simulink model "quad_copter_ct_dt"  (R2016a)
settings: Solver=VariableStepAuto  StartTime=0.0  StopTime=10.0  RelTol=1e-3
undefined symbols (not defined in the file): DiscIntNeverNeededParam, Mixer, PitchRateModel_dt, PitchRateModel_tf, Ri_dt, Ri_tf, Ro_dt, Ro_tf, Ts
settings Model: Creator=tibo  LastModifiedBy=tibo

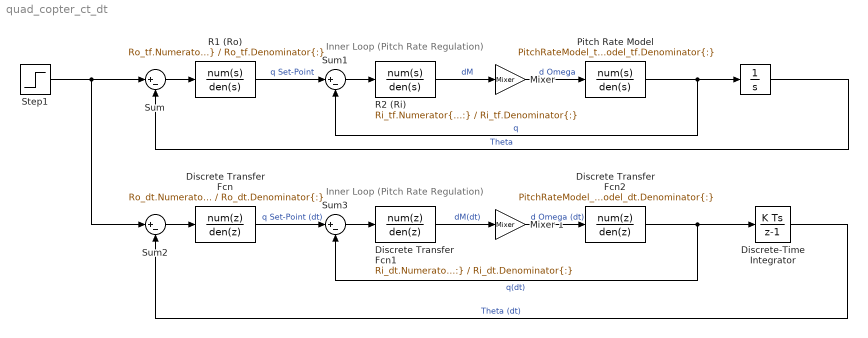
== system quad_copter_ct_dt ==
  note: Inner Loop (Pitch Rate Regulation)
  note: Inner Loop (Pitch Rate Regulation)
  " " : Integrator  ContinuousStateAttributes='PitchAngle'
  Discrete Transfer Fcn : DiscreteTransferFcn  Numerator=Ro_dt.Numerator{:}  Denominator=Ro_dt.Denominator{:}  SampleTime=Ts
  Discrete Transfer Fcn1 : DiscreteTransferFcn  Numerator=Ri_dt.Numerator{:}  Denominator=Ri_dt.Denominator{:}
  Discrete Transfer Fcn2 : DiscreteTransferFcn  Numerator=PitchRateModel_dt.Numerator{:}  Denominator=PitchRateModel_dt.Denominator{:}
  Discrete-Time Integrator : DiscreteIntegrator  InitialConditionSetting=State (most efficient)  ICPrevOutput=DiscIntNeverNeededParam  ICPrevScaledInput=DiscIntNeverNeededParam
  "Mixer " : Gain  Gain=Mixer
  Mixer 1 : Gain  Gain=Mixer
  "Pitch Rate Model " : TransferFcn  Numerator=PitchRateModel_tf.Numerator{:}  Denominator=PitchRateModel_tf.Denominator{:}  ContinuousStateAttributes='PitchRate'
  "R1 (Ro) " : TransferFcn  Numerator=Ro_tf.Numerator{:}  Denominator=Ro_tf.Denominator{:}
  "R2 (Ri) " : TransferFcn  Numerator=Ri_tf.Numerator{:}  Denominator=Ri_tf.Denominator{:}
  Step1 : Step  After=.18  SampleTime=0
  Sum{,1..3} (4 alike) : Sum  Inputs=|+-
  wires:
  Sum/1 -> "R1 (Ro) "/1
  "R1 (Ro) "/1 -> Sum1/1  "q Set-Point"
  "R2 (Ri) "/1 -> "Mixer "/1  "dM"
  "Mixer "/1 -> "Pitch Rate Model "/1  "d Omega"
  "Pitch Rate Model "/1 -> Sum1/2, " "/1  "q"
  " "/1 -> Sum/2  "Theta"
  Sum1/1 -> "R2 (Ri) "/1
  Step1/1 -> Sum2/1, Sum/1
  Sum2/1 -> Discrete Transfer Fcn/1
  Discrete Transfer Fcn/1 -> Sum3/1  "q Set-Point (dt)"
  Discrete Transfer Fcn1/1 -> Mixer 1/1  "dM(dt)"
  Mixer 1/1 -> Discrete Transfer Fcn2/1  "d Omega (dt)"
  Discrete Transfer Fcn2/1 -> Discrete-Time Integrator/1, Sum3/2  "q(dt)"
  Discrete-Time Integrator/1 -> Sum2/2  "Theta (dt)"
  Sum3/1 -> Discrete Transfer Fcn1/1
